simulink model "inverse_control"  (R2020a)
settings: Solver=VariableStepAuto  StartTime=0.0  StopTime=700  RelTol=1e-3
undefined symbols (not defined in the file): C, W
libraries: simulink x2
settings Model: Creator=elkin  LastModifiedBy=elkin

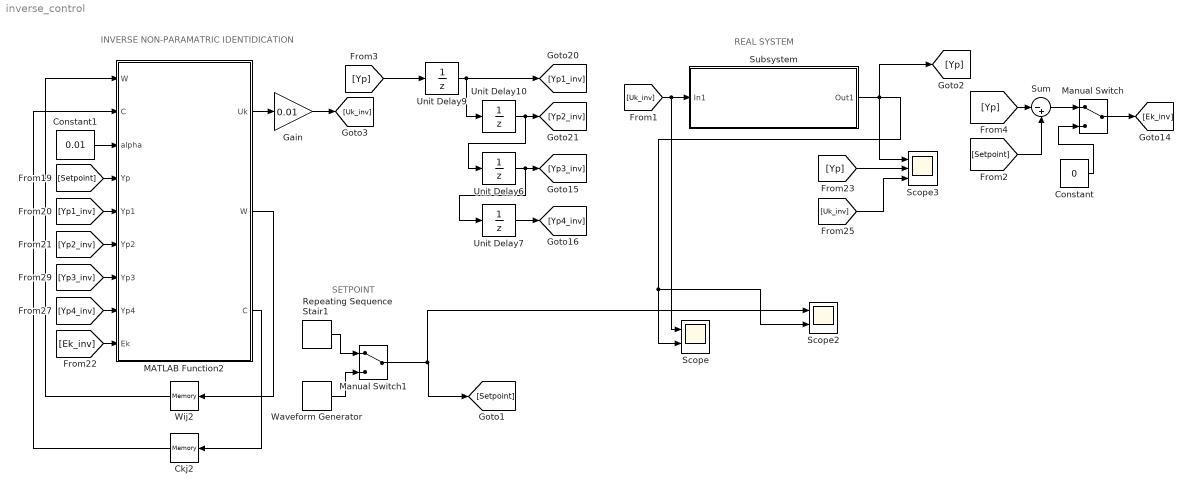
== system inverse_control ==
  note: SETPOINT
  note: REAL SYSTEM
  note: INVERSE NON-PARAMATRIC IDENTIDICATION
  Ckj2 : Memory  InitialCondition=C
  Constant : Constant  Value=0
  Constant1 : Constant  Value=0.01
  Gain : Gain  Gain=0.01
  MATLAB Function2 : MATLAB Function  TreatAsAtomicUnit=on
  Manual Switch : ManualSwitch
  Manual Switch1 : ManualSwitch
  Repeating Sequence Stair1 : simulink/Sources/Repeating Sequence Stair  OutValues=[0 0.2 0 0.4 0.8 0.4 1].'  tsamp=50  OutMin=[]  OutMax=[]  OutDataTypeStr=double  OutputDataTypeScalingMode=double  OutDataType=fixdt(0,8)  ConRadixGroup=Best Precision: Vector-wise  OutScaling=2^-12
  Scope : Scope  NumInputPorts=2
  Scope2 : Scope  NumInputPorts=2
  Scope3 : Scope  NumInputPorts=3
  Subsystem : Subsystem
  Sum : Sum  Inputs=|-+
  Unit Delay{6..7,9..10} (4 alike) : UnitDelay  SampleTime=-1  HasFrameUpgradeWarning=on
  Waveform Generator : simulink/Sources/Waveform Generator  OutMin=[]  OutMax=[]  OutDataTypeStr=double  SelectedSignal=1  Signals=sin(1, 0.03, 0)  BlockNames=MultiportSwitch_45ff84b921fe4c9  SampleTime=0.1
  Wij2 : Memory  InitialCondition=W
  wires:
  Subsystem/1(Out1) -> [Yp], Scope3/1, Scope2/2, Scope/2
  Constant/1 -> Manual Switch/2
  [Uk_inv] -> Scope3/3
  [Yp3_inv] -> MATLAB Function2/7(Yp3)
  MATLAB Function2/2(W) -> Wij2/1
  [Yp4_inv] -> MATLAB Function2/8(Yp4)
  MATLAB Function2/3(C) -> Ckj2/1
  [Setpoint] -> MATLAB Function2/4(Yp)
  [Yp1_inv] -> MATLAB Function2/5(Yp1)
  [Yp2_inv] -> MATLAB Function2/6(Yp2)
  Constant1/1 -> MATLAB Function2/3(alpha)
  Ckj2/1 -> MATLAB Function2/2("C ")
  MATLAB Function2/1(Uk) -> Gain/1
  [Yp] -> Scope3/2
  [Uk_inv] -> Scope/1, Subsystem/1(In1)
  Repeating Sequence Stair1/1 -> Manual Switch1/1
  Waveform Generator/1 -> Manual Switch1/2
  Manual Switch1/1 -> Scope2/1, [Setpoint]
  [Setpoint] -> Sum/2
  Sum/1 -> Manual Switch/1
  Manual Switch/1 -> [Ek_inv]
  Wij2/1 -> MATLAB Function2/1("W ")
  [Ek_inv] -> MATLAB Function2/9(Ek)
  Unit Delay6/1 -> Unit Delay7/1, [Yp3_inv]
  [Yp] -> Unit Delay9/1
  Unit Delay10/1 -> Unit Delay6/1, [Yp2_inv]
  Unit Delay7/1 -> [Yp4_inv]
  Unit Delay9/1 -> [Yp1_inv], Unit Delay10/1
  [Yp] -> Sum/1
  Gain/1 -> [Uk_inv]

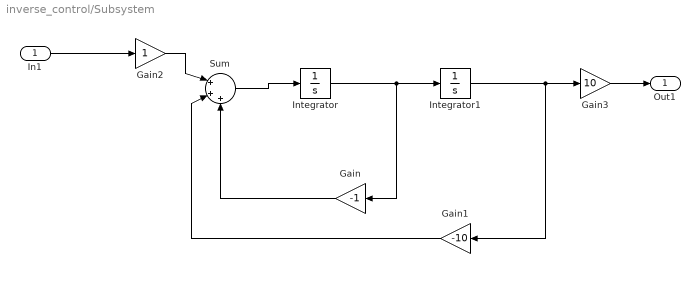
== system inverse_control/Subsystem ==
  In1 : Inport
  Gain : Gain  Gain=-1
  Gain1 : Gain  Gain=-10
  Gain2 : Gain
  Gain3 : Gain  Gain=10
  Integrator : Integrator
  Integrator1 : Integrator
  Sum : Sum  Inputs=|+++
  Out1 : Outport  VectorParamsAs1DForOutWhenUnconnected=off
  wires:
  Integrator/1 -> Gain/1, Integrator1/1
  Gain2/1 -> Sum/1
  Gain1/1 -> Sum/2
  Sum/1 -> Integrator/1
  Integrator1/1 -> Gain3/1, Gain1/1
  Gain/1 -> Sum/3
  In1/1 -> Gain2/1
  Gain3/1 -> Out1/1

== matlab function inverse_control/MATLAB Function2 ==
  data: W input; Uk output; C input; alpha input; Yp input; Yp1 input; Yp2 input; Yp3 input; Yp4 input; Ek input; W output; C output
function [Uk, W, C] = fcn(W, C, alpha, Yp, Yp1, Yp2, Yp3, Yp4, Ek)
    % Define input vector
    X = [Yp Yp1 Yp2 Yp3 Yp4];
    
    % Calculate Aj in the hidden layer
    Aj = W*X';
    
    % Activation function of the hidden layer
    H = tanh(Aj);
    
    % Calculate Ak in the output layer
    Ak = C'*H;
    
    % Activation function of the output layer
    Uk = Ak;
    
    % Update C matrix
    C = C + alpha*Ek*H;
    
    % Update W matrix
    Hd = sech(Aj).^2;
    W = W + alpha*Ek*(C.*Hd)*X;
